simulink model "MEEN_432_Proj1Part1"  (R2025a)
settings: Solver=VariableStepAuto  StartTime=0.0  StopTime=25  RelTol=1e-3
model workspace (MATLAB code in the model file):
  | time_step = 1
libraries: simulink x1
settings Model: NumberOfSteps=100  Creator=caleb  LastModifiedBy=caleb

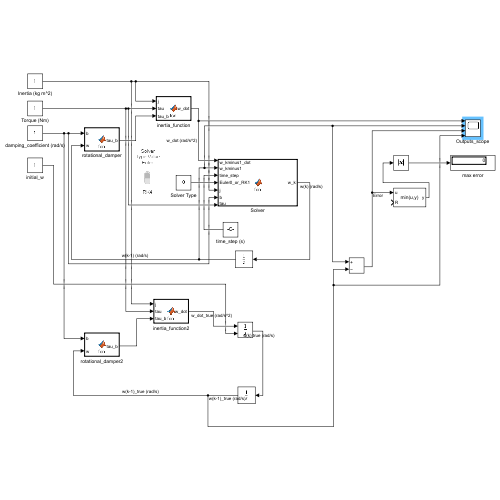
[thumbnail: Simulink's stored preview of the top-level diagram]
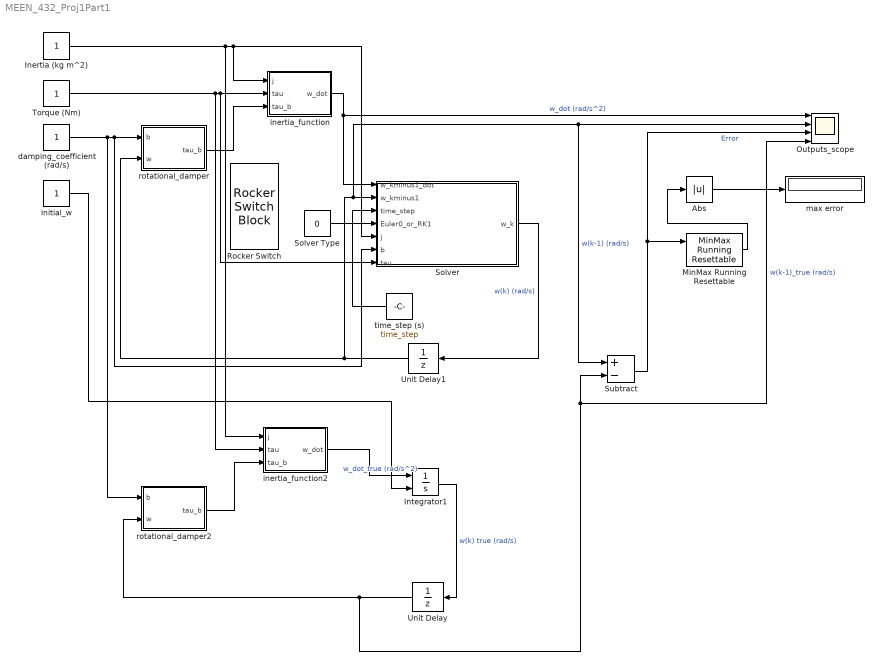
== system MEEN_432_Proj1Part1 ==
  Abs : Abs  SaturateOnIntegerOverflow=off
  Inertia (kg m^2) : Constant
  Integrator1 : Integrator  InitialConditionSource=external  InitialCondition=-1
  MinMax Running Resettable : simulink/Math Operations/MinMax Running Resettable  Function=min  vinit=0.0
  Outputs_scope : Scope  NumInputPorts=4
      settings: ActiveDisplayYMinimum=-12.662603834949234  ActiveDisplayYMaximum=23.951630640983275
  Rocker Switch : RockerSwitchBlock
  Solver : MATLAB Function  TreatAsAtomicUnit=on
  Solver Type : Constant  Value=0
  Subtract : Sum  Inputs=+-
  Torque (Nm) : Constant
  Unit Delay : UnitDelay  InitialCondition=1  SampleTime=0.001  HasFrameUpgradeWarning=on
  Unit Delay1 : UnitDelay  InitialCondition=1  SampleTime=-1  HasFrameUpgradeWarning=on
  damping_coefficient (rad/s) : Constant
  inertia_function : MATLAB Function  TreatAsAtomicUnit=on
  inertia_function2 : MATLAB Function  TreatAsAtomicUnit=on
  initial_w : Constant
  max error : Display
  rotational_damper : MATLAB Function  TreatAsAtomicUnit=on
  rotational_damper2 : MATLAB Function  TreatAsAtomicUnit=on
  time_step (s) : Constant  Value=time_step  SampleTime=time_step
  wires:
  inertia_function/1(w_dot) -> Solver/1(w_kminus1_dot), Outputs_scope/1  "w_dot (rad/s^2)"
  Solver/1(w_k) -> Unit Delay1/1  "w(k) (rad/s)"
  rotational_damper/1(tau_b) -> inertia_function/3(tau_b)
  Unit Delay1/1 -> rotational_damper/2(w), Subtract/1, Outputs_scope/2, Solver/2(w_kminus1)  "w(k-1) (rad/s)"
  Solver Type/1 -> Solver/4(Euler0_or_RK1)
  time_step (s)/1 -> Solver/3(time_step)
  inertia_function2/1(w_dot) -> Integrator1/1  "w_dot_true (rad/s^2)"
  Inertia (kg m^2)/1 -> inertia_function2/1(j), inertia_function/1(j), Solver/5(j)
  rotational_damper2/1(tau_b) -> inertia_function2/3(tau_b)
  Integrator1/1 -> Unit Delay/1  "w(k) true (rad/s)"
  Torque (Nm)/1 -> inertia_function2/2(tau), Solver/7(tau), inertia_function/2(tau)
  damping_coefficient (rad/s)/1 -> Solver/6(b), rotational_damper/1(b), rotational_damper2/1(b)
  Subtract/1 -> Outputs_scope/3, MinMax Running Resettable/1  "Error"
  Unit Delay/1 -> Subtract/2, Outputs_scope/4, rotational_damper2/2(w)  "w(k-1)_true (rad/s)"
  initial_w/1 -> Integrator1/2
  MinMax Running Resettable/1 -> Abs/1
  Abs/1 -> max error/1

== matlab function MEEN_432_Proj1Part1/rotational_damper ==
  data: b input; tau_b output; w input
function tau_b = fcn(b, w)

tau_b = b*w;

== matlab function MEEN_432_Proj1Part1/inertia_function ==
  data: j input; w_dot output; tau input; tau_b input
function w_dot = fcn(j, tau, tau_b)


w_dot = (1/j)*(tau - tau_b);

== matlab function MEEN_432_Proj1Part1/Solver ==
  data: w_kminus1_dot input; w_k output; w_kminus1 input; time_step input; Euler0_or_RK1 input; j input; b input; tau input
function w_k  = fcn(w_kminus1_dot, w_kminus1, time_step, Euler0_or_RK1, j, b, tau)
if Euler0_or_RK1 == 1;
    w_k = w_kminus1 + w_kminus1_dot*time_step;
    
elseif Euler0_or_RK1 == 0;
    k1 = w_kminus1_dot;
    k2 = (1/j)*(tau - ((w_kminus1 + k1*time_step/2)*b));
    k3 = (1/j)*(tau - ((w_kminus1 + k2*time_step/2)*b));
    k4 = (1/j)*(tau - ((w_kminus1 + k3*time_step)*b));

    w_k = w_kminus1 + (1/6)*(k1 + 2*k2 + 2*k3 + k4)*time_step;

else
    w_k = 0;

end

== matlab function MEEN_432_Proj1Part1/inertia_function2 ==
  data: j input; w_dot output; tau input; tau_b input
function w_dot = fcn(j, tau, tau_b)


w_dot = (1/j)*(tau - tau_b);

== matlab function MEEN_432_Proj1Part1/rotational_damper2 ==
  data: b input; tau_b output; w input
function tau_b = fcn(b, w)

tau_b = b*w;
